simulink library "Hexarotor_HIL"  (R2026a)
settings: Solver=VariableStepAuto
settings Model: Creator=Yuhao  LastModifiedBy=Yuhao

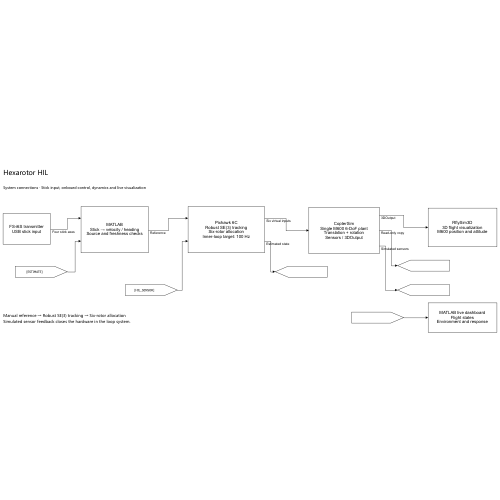
[thumbnail: Simulink's stored preview of the top-level diagram]
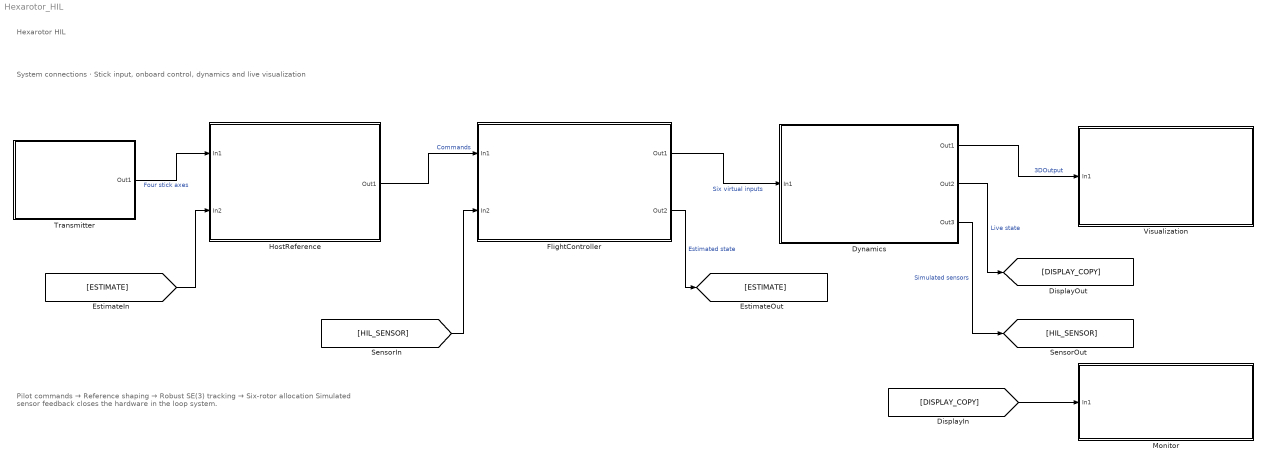
== system Hexarotor_HIL ==
  note: Hexarotor HIL
  note: System connections · Stick input, onboard control, dynamics and live visualization
  note: Pilot commands → Reference shaping → Robust SE(3) tracking → Six-rotor allocation
      | Simulated sensor feedback closes the hardware in the loop system.
  Dynamics : Subsystem
      mask Display: disp(sprintf('CopterSim\nSingle M600 6-DoF plant\nTranslation + rotation\nSensors / 3DOutput'))
  FlightController : Subsystem
      mask Display: disp(sprintf('Pixhawk 6C\nReference shaping\nRobust SE(3) tracking\nSix-rotor allocation'))
  HostReference : Subsystem
      mask Display: disp(sprintf('MATLAB\nCommand processing\nVelocity and yaw rate'))
  Monitor : Subsystem
      mask Display: disp(sprintf('MATLAB live dashboard\nFlight states\nEnvironment and response'))
  Transmitter : Subsystem
      mask Display: disp(sprintf('FS-i6S transmitter\nUSB stick input'))
  Visualization : Subsystem
      mask Display: disp(sprintf('RflySim3D\n3D flight visualization\nM600 position and attitude'))
  wires:
  Transmitter/1(Out1) -> HostReference/1(In1)  "Four stick axes"
  HostReference/1(Out1) -> FlightController/1(In1)  "Commands"
  FlightController/1(Out1) -> Dynamics/1(In1)  "Six virtual inputs"
  Dynamics/1(Out1) -> Visualization/1(In1)  "3DOutput"
  FlightController/2(Out2) -> [ESTIMATE]  "Estimated state"
  [ESTIMATE] -> HostReference/2(In2)
  Dynamics/3(Out3) -> [HIL_SENSOR]  "Simulated sensors"
  [HIL_SENSOR] -> FlightController/2(In2)
  Dynamics/2(Out2) -> [DISPLAY_COPY]  "Live state"
  [DISPLAY_COPY] -> Monitor/1(In1)

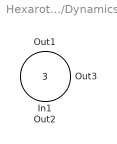
== system Hexarotor_HIL/Dynamics ==
  In1 : Inport
  Out1 : Outport
  Out2 : Outport  Port=2
  Out3 : Outport  Port=3

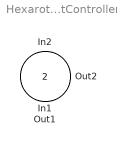
== system Hexarotor_HIL/FlightController ==
  In1 : Inport
  In2 : Inport  Port=2
  Out1 : Outport
  Out2 : Outport  Port=2

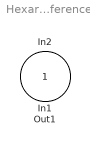
== system Hexarotor_HIL/HostReference ==
  In1 : Inport
  In2 : Inport  Port=2
  Out1 : Outport

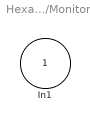
== system Hexarotor_HIL/Monitor ==
  In1 : Inport

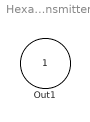
== system Hexarotor_HIL/Transmitter ==
  Out1 : Outport

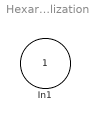
== system Hexarotor_HIL/Visualization ==
  In1 : Inport
